simulink model "ThyroidCheckupV2"  (R2022a)
settings: Solver=VariableStepAuto  StartTime=0.0  StopTime=10.0  RelTol=1e-3
settings Model: Creator=NEMALI MAHESH  LastModifiedBy=NEMALI MAHESH

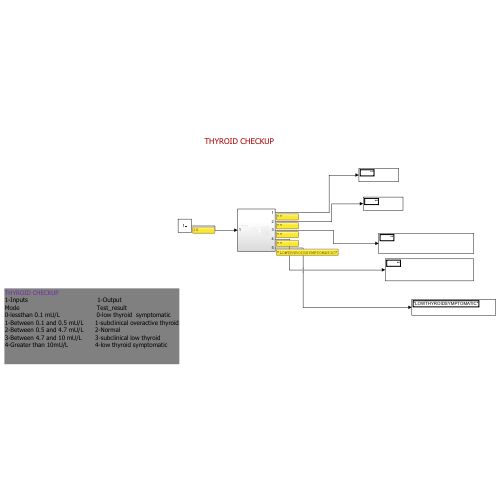
[thumbnail: Simulink's stored preview of the top-level diagram]
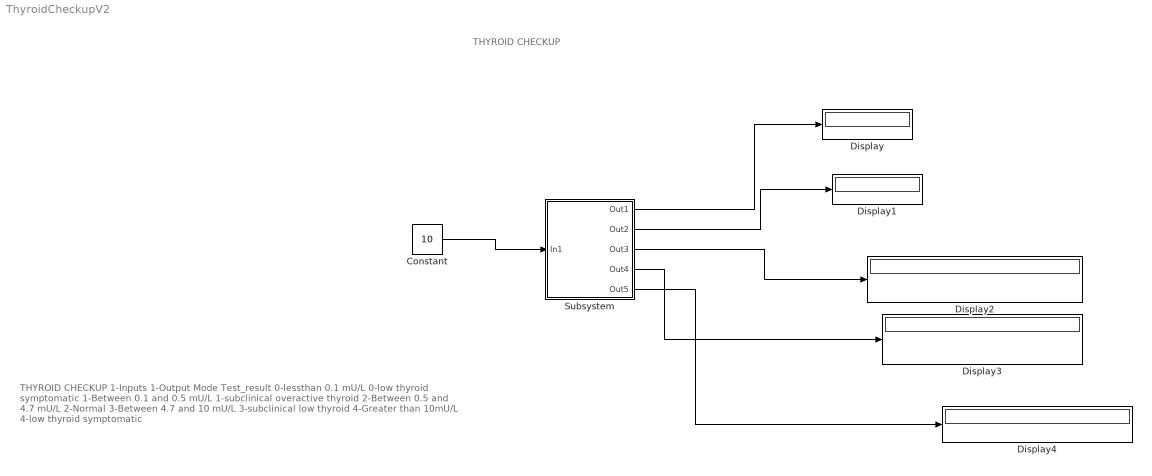
== system ThyroidCheckupV2 ==
  note: THYROID CHECKUP
  note: THYROID CHECKUP
      | 1-Inputs 1-Output
      | Mode Test_result
      | 0-lessthan 0.1 mU/L 0-low thyroid symptomatic
      | 1-Between 0.1 and 0.5 mU/L 1-subclinical overactive thyroid
      | 2-Between 0.5 and 4.7 mU/L 2-Normal
      | 3-Between 4.7 and 10 mU/L 3-subclinical low thyroid
      | 4-Greater than 10mU/L 4-low thyroid symptomatic
  Constant : Constant  Value=10
  Display{,1..4} (5 alike) : Display
  Subsystem : Subsystem
  wires:
  Constant/1 -> Subsystem/1(In1)
  Subsystem/1(Out1) -> Display/1
  Subsystem/2(Out2) -> Display1/1
  Subsystem/3(Out3) -> Display2/1
  Subsystem/4(Out4) -> Display3/1
  Subsystem/5(Out5) -> Display4/1

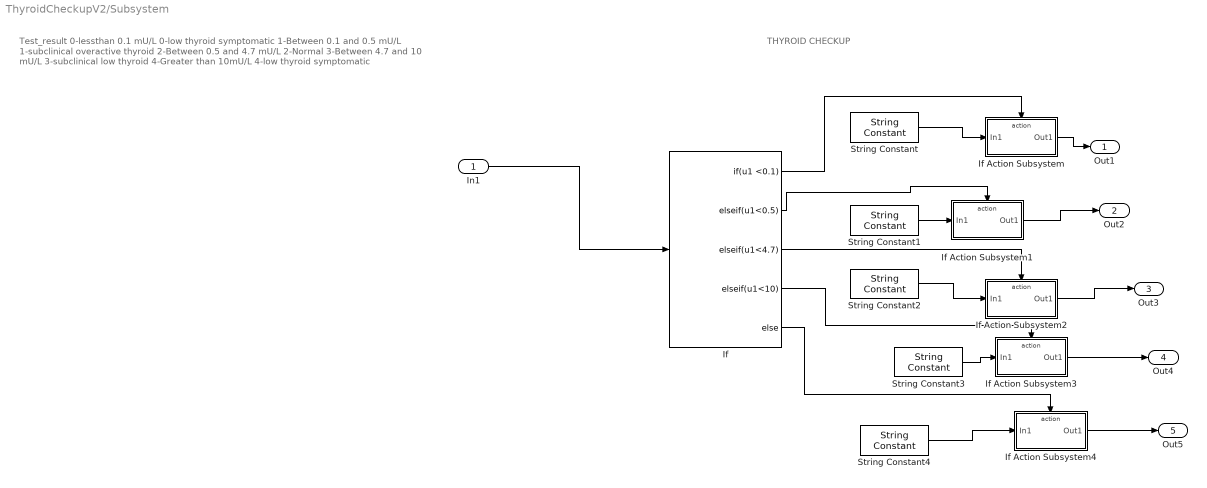
== system ThyroidCheckupV2/Subsystem ==
  note: Test_result
      | 0-lessthan 0.1 mU/L 0-low thyroid symptomatic
      | 1-Between 0.1 and 0.5 mU/L 1-subclinical overactive thyroid
      | 2-Between 0.5 and 4.7 mU/L 2-Normal
      | 3-Between 4.7 and 10 mU/L 3-subclinical low thyroid
      | 4-Greater than 10mU/L 4-low thyroid symptomatic
  note: THYROID CHECKUP
  In1 : Inport
  If : If  IfExpression=u1 <0.1  ElseIfExpressions=u1<0.5,u1<4.7,u1<10
  If Action Subsystem : Subsystem  TreatAsAtomicUnit=on
  If Action Subsystem1 : Subsystem  TreatAsAtomicUnit=on
  If Action Subsystem2 : Subsystem  TreatAsAtomicUnit=on
  If Action Subsystem3 : Subsystem  TreatAsAtomicUnit=on
  If Action Subsystem4 : Subsystem  TreatAsAtomicUnit=on
  String Constant : StringConstant  String="\"LOW THYROID SYMPTOMATIC\""
  String Constant1 : StringConstant  String="\"SUBCLINICAL OVERACTIVE \""
  String Constant2 : StringConstant  String="\"NORMAL\""
  String Constant3 : StringConstant  String="\"SUBCLINICAL LOW THYROID\""
  String Constant4 : StringConstant  String="\"LOWTHYROIDSYMPTOMATIC\""
  Out1 : Outport
  Out2 : Outport  Port=2
  Out3 : Outport  Port=3
  Out4 : Outport  Port=4
  Out5 : Outport  Port=5
  wires:
  If/4 -> If Action Subsystem3/Action
  If/3 -> If Action Subsystem2/Action
  If/1 -> If Action Subsystem/Action
  If/5 -> If Action Subsystem4/Action
  String Constant/1 -> If Action Subsystem/1(In1)
  String Constant4/1 -> If Action Subsystem4/1(In1)
  If Action Subsystem2/1(Out1) -> Out3/1
  In1/1 -> If/1
  If/2 -> If Action Subsystem1/Action
  If Action Subsystem/1(Out1) -> Out1/1
  If Action Subsystem4/1(Out1) -> Out5/1
  If Action Subsystem3/1(Out1) -> Out4/1
  If Action Subsystem1/1(Out1) -> Out2/1
  String Constant1/1 -> If Action Subsystem1/1(In1)
  String Constant2/1 -> If Action Subsystem2/1(In1)
  String Constant3/1 -> If Action Subsystem3/1(In1)

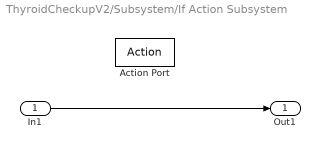
== system ThyroidCheckupV2/Subsystem/If Action Subsystem ==
  In1 : Inport
  Action Port : ActionPort  ActionPortLabel=if(u1 <0.1)
  Out1 : Outport
  wires:
  In1/1 -> Out1/1

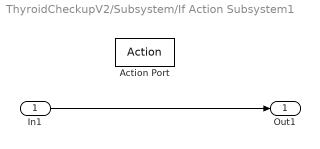
== system ThyroidCheckupV2/Subsystem/If Action Subsystem1 ==
  In1 : Inport
  Action Port : ActionPort  ActionPortLabel=elseif(u1<0.5)
  Out1 : Outport
  wires:
  In1/1 -> Out1/1

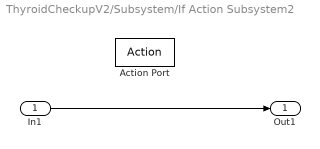
== system ThyroidCheckupV2/Subsystem/If Action Subsystem2 ==
  In1 : Inport
  Action Port : ActionPort  ActionPortLabel=elseif(u1<4.7)
  Out1 : Outport
  wires:
  In1/1 -> Out1/1

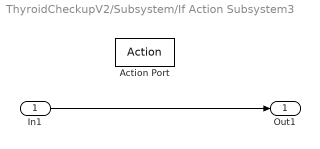
== system ThyroidCheckupV2/Subsystem/If Action Subsystem3 ==
  In1 : Inport
  Action Port : ActionPort  ActionPortLabel=elseif(u1<10)
  Out1 : Outport
  wires:
  In1/1 -> Out1/1

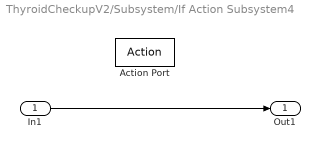
== system ThyroidCheckupV2/Subsystem/If Action Subsystem4 ==
  In1 : Inport
  Action Port : ActionPort  ActionPortLabel=else
  Out1 : Outport
  wires:
  In1/1 -> Out1/1
